simulink model "test1"  (R2020a)
settings: Solver=VariableStepAuto  StartTime=0.0  StopTime=inf  FixedStep=Ts  RelTol=1e-3
PostLoadFcn:
  | , if any(exist('dsrtsu_mdlpostloadfcn', 'file') ~= 0), dsrtsu_mdlpostloadfcn('Execute', bdroot); end,
InitFcn:
  | , if any(exist('rtifpga_mdlclblib', 'file') ~= 0), rtifpga_mdlclblib('Init', bdroot); end,
model workspace (MAT data in the model file):
  FPGA_test1_1_Interrupt_1_1_write : Simulink.Signal (value not decoded)
  FPGA_test1_1_Register_1_1_1_write : Simulink.Signal (value not decoded)
  FPGA_test1_1_Register_2_1_1_write : Simulink.Signal (value not decoded)
  FPGA_test1_1_Register_3_1_1_write : Simulink.Signal (value not decoded)
  FPGA_test1_1_Register_4_1_1_write : Simulink.Signal (value not decoded)
values from neighbouring files (symbols this model uses):
  clamp_threshold = 200    [param.m]
  io_fixed_gain = 10*1000/(3*100)    (= 33.3333333333)    [param.m]
  io_sonda_gain = 10/0.010    (= 1000)    [param.m]
  ioa_gain = 1    [param.m]
  ioa_offset = 0.12    [param.m]
  iob_gain = 1    [param.m]
  iob_offset = 0.06    [param.m]
  ioc_gain = 1    [param.m]
  ioc_offset = -0.1    [param.m]
  Ts = 20e-6    (= 2e-05)    [param.m]
  vclamp_gain = 1010    [param.m]
  vclamp_offset = 10.5    [param.m]
  vi_fixed_gain = 10*44    (= 440)    [param.m]
  vi_sonda_gain = 10*200    (= 2000)    [param.m]
  via_gain = 1    [param.m]
  via_offset = 2.2    [param.m]
  vib_gain = 1    [param.m]
  vib_offset = 3    [param.m]
  vic_gain = 1    [param.m]
  vic_offset = 4.2    [param.m]
libraries: xbsIndex_r4 x428, rti1202lib_adc_class1 x9, rtiproclib x6, simulink x2, rtifpgainterfacelib x1
(part 6 of 7)

== system test1/4_step/FPGA_XDATA_READ_BL1 ==
  CEP1 : xbsIndex_r4/Clock Enable Probe  inherit_constraints=off  block_type=ceprobe
      settings: infoedit="Clock enable extractor.  Produces a Boolean output that mirrors the hardware clock enable associated with the input sample rate.<br><br>Hardware notes: in hardware this block costs nothing."
  CEP3 : xbsIndex_r4/Clock Enable Probe  inherit_constraints=off  block_type=ceprobe
      settings: infoedit="Clock enable extractor.  Produces a Boolean output that mirrors the hardware clock enable associated with the input sample rate.<br><br>Hardware notes: in hardware this block costs nothing."
  Constant1 : xbsIndex_r4/Constant  const=1  gui_display_data_type=Fixed-point  arith_type=Boolean  n_bits=16  bin_pt=14  preci_type=Single  exp_width=8  frac_width=24  explicit_period=on  period=1*1e-08  equ=P=C  opselect=C  inp2=PCIN>>17  opr=+  inp1=P  carry=CIN  dbl_ovrd=off  block_type=constant
  Constant3 : xbsIndex_r4/Constant  const=1  gui_display_data_type=Fixed-point  arith_type=Boolean  n_bits=16  bin_pt=14  preci_type=Single  exp_width=8  frac_width=24  explicit_period=on  period=1*1e-08  equ=P=C  opselect=C  inp2=PCIN>>17  opr=+  inp1=P  carry=CIN  dbl_ovrd=off  block_type=constant
  Delay1 : xbsIndex_r4/Delay  rst=off  infoeditControl=Selection of Reset will increase slice count due to use of real FFs and instead of SRLs  en=off  latency=0  reg_retiming=off  dbl_ovrd=off  block_type=delay
  Delay3 : xbsIndex_r4/Delay  rst=off  infoeditControl=Selection of Reset will increase slice count due to use of real FFs and instead of SRLs  en=off  latency=0  reg_retiming=off  dbl_ovrd=off  block_type=delay
  Register1 : xbsIndex_r4/Register  init=0  rst=off  en=on  dbl_ovrd=off  block_type=register
  Register3 : xbsIndex_r4/Register  init=0  rst=off  en=on  dbl_ovrd=off  block_type=register
  phs_read_register : Subsystem
      mask init:
      | [par, fct] = rtifpgafcnlib('GetCurrentParaValue', get_param(get(gcbh, 'parent'), 'handle'), 'all');
      | if isempty(par) || isempty(fct)
      |     return
      | end
      | binaryPoint = str2double(par(1).Value{1});
      | format = par(2).Value{1};
      | if (strcmp(format, 'signed') == 1)
      |     mode = 0;
      | elseif (strcmp(format, 'unsigned') == 1)
      |     mode = 1;
      | else
      |     % floating-point
      |     mode = 2;
      | end
      | 
      | %Determine PROC sample time
      | proc_sample_time_field = par(5).Value{1};
      | num_val = str2num(proc_sample_time_field);
      | if ~isempty(num_val)
      |     proc_sample_time = num_val;
      | else % search for subsystem/workspace value
      |     proc_sample_time = rtifpgafcnlib('SearchVariableValue', gcbh, proc_sample_time_field);
      |     if ~isnumeric(proc_sample_time)
      |         proc_sample_time = str2double(proc_sample_time);
      |     end
      | end
      | 
      | %Determine FPGA sample rate
      | dataGatewayName = fct.FrameworkIn(1).Name{1};
      | fpga_sample_time = rtifpga_xsgcasinglib('xlGetParam', [gcs '/' dataGatewayName] , 'period');
      | fpga_sample_time = str2double(fpga_sample_time);
  xreg_000_dout : xbsIndex_r4/Gateway In  gui_display_data_type=Fixed-point  arith_type=Unsigned  n_bits=32  bin_pt=0  preci_type=Single  exp_width=8  frac_width=24  rows=1  columns=1  quantization="Round  (unbiased: +/- Inf)"  overflow=Saturate  period=1e-08  UseAsADC=off  ADCChannel='1'  interface=None  automatic_assignment=on  address_offset=hex2dec('00')  intf_name=''  intf_description=''  default_value=0  timing_constraint=None  locs_specified=off  LOCs={}  io_standard={}  inherit_from_input=off  hdl_port=on  dbl_ovrd=off  block_type=gatewayin
  xreg_000_dout_wr : xbsIndex_r4/Gateway In  gui_display_data_type=Fixed-point  arith_type=Unsigned  n_bits=1  bin_pt=0  preci_type=Single  exp_width=8  frac_width=24  rows=1  columns=1  quantization="Round  (unbiased: +/- Inf)"  overflow=Saturate  period=1e-08  UseAsADC=off  ADCChannel='1'  interface=None  automatic_assignment=on  address_offset=hex2dec('00')  intf_name=''  intf_description=''  default_value=0  timing_constraint=None  locs_specified=off  LOCs={}  io_standard={}  inherit_from_input=off  hdl_port=on  dbl_ovrd=off  block_type=gatewayin
  Data : Outport
  Data New : Outport  Port=2
  wires:
  [FPGA_test1_1_Register_1_1_1_write] -> phs_read_register/1(data_i)
  Register1/1 -> Delay1/1
  Delay1/1 -> Data/1
  Constant1/1 -> CEP1/1
  CEP1/1 -> Register1/2
  xreg_000_dout/1 -> Register1/1
  Register3/1 -> Delay3/1
  Delay3/1 -> Data New/1
  Constant3/1 -> CEP3/1
  CEP3/1 -> Register3/2
  xreg_000_dout_wr/1 -> Register3/1
  phs_read_register/1(data_o) -> xreg_000_dout/1
  phs_read_register/2(data_new_o) -> xreg_000_dout_wr/1

== system test1/4_step/FPGA_XDATA_READ_BL2 ==
  CEP1 : xbsIndex_r4/Clock Enable Probe  inherit_constraints=off  block_type=ceprobe
      settings: infoedit="Clock enable extractor.  Produces a Boolean output that mirrors the hardware clock enable associated with the input sample rate.<br><br>Hardware notes: in hardware this block costs nothing."
  CEP3 : xbsIndex_r4/Clock Enable Probe  inherit_constraints=off  block_type=ceprobe
      settings: infoedit="Clock enable extractor.  Produces a Boolean output that mirrors the hardware clock enable associated with the input sample rate.<br><br>Hardware notes: in hardware this block costs nothing."
  Constant1 : xbsIndex_r4/Constant  const=1  gui_display_data_type=Fixed-point  arith_type=Boolean  n_bits=16  bin_pt=14  preci_type=Single  exp_width=8  frac_width=24  explicit_period=on  period=1*1e-08  equ=P=C  opselect=C  inp2=PCIN>>17  opr=+  inp1=P  carry=CIN  dbl_ovrd=off  block_type=constant
  Constant3 : xbsIndex_r4/Constant  const=1  gui_display_data_type=Fixed-point  arith_type=Boolean  n_bits=16  bin_pt=14  preci_type=Single  exp_width=8  frac_width=24  explicit_period=on  period=1*1e-08  equ=P=C  opselect=C  inp2=PCIN>>17  opr=+  inp1=P  carry=CIN  dbl_ovrd=off  block_type=constant
  Delay1 : xbsIndex_r4/Delay  rst=off  infoeditControl=Selection of Reset will increase slice count due to use of real FFs and instead of SRLs  en=off  latency=0  reg_retiming=off  dbl_ovrd=off  block_type=delay
  Delay3 : xbsIndex_r4/Delay  rst=off  infoeditControl=Selection of Reset will increase slice count due to use of real FFs and instead of SRLs  en=off  latency=0  reg_retiming=off  dbl_ovrd=off  block_type=delay
  Register1 : xbsIndex_r4/Register  init=0  rst=off  en=on  dbl_ovrd=off  block_type=register
  Register3 : xbsIndex_r4/Register  init=0  rst=off  en=on  dbl_ovrd=off  block_type=register
  phs_read_register : Subsystem
      mask init: same as test1/4_step/FPGA_XDATA_READ_BL1/phs_read_register
  xreg_001_dout : xbsIndex_r4/Gateway In  gui_display_data_type=Fixed-point  arith_type=Unsigned  n_bits=32  bin_pt=0  preci_type=Single  exp_width=8  frac_width=24  rows=1  columns=1  quantization="Round  (unbiased: +/- Inf)"  overflow=Saturate  period=1e-08  UseAsADC=off  ADCChannel='1'  interface=None  automatic_assignment=on  address_offset=hex2dec('00')  intf_name=''  intf_description=''  default_value=0  timing_constraint=None  locs_specified=off  LOCs={}  io_standard={}  inherit_from_input=off  hdl_port=on  dbl_ovrd=off  block_type=gatewayin
  xreg_001_dout_wr : xbsIndex_r4/Gateway In  gui_display_data_type=Fixed-point  arith_type=Unsigned  n_bits=1  bin_pt=0  preci_type=Single  exp_width=8  frac_width=24  rows=1  columns=1  quantization="Round  (unbiased: +/- Inf)"  overflow=Saturate  period=1e-08  UseAsADC=off  ADCChannel='1'  interface=None  automatic_assignment=on  address_offset=hex2dec('00')  intf_name=''  intf_description=''  default_value=0  timing_constraint=None  locs_specified=off  LOCs={}  io_standard={}  inherit_from_input=off  hdl_port=on  dbl_ovrd=off  block_type=gatewayin
  Data : Outport
  Data New : Outport  Port=2
  wires:
  [FPGA_test1_1_Register_2_1_1_write] -> phs_read_register/1(data_i)
  Register1/1 -> Delay1/1
  Delay1/1 -> Data/1
  Constant1/1 -> CEP1/1
  CEP1/1 -> Register1/2
  xreg_001_dout/1 -> Register1/1
  Register3/1 -> Delay3/1
  Delay3/1 -> Data New/1
  Constant3/1 -> CEP3/1
  CEP3/1 -> Register3/2
  xreg_001_dout_wr/1 -> Register3/1
  phs_read_register/1(data_o) -> xreg_001_dout/1
  phs_read_register/2(data_new_o) -> xreg_001_dout_wr/1

== system test1/4_step/FPGA_XDATA_READ_BL3 ==
  CEP1 : xbsIndex_r4/Clock Enable Probe  inherit_constraints=off  block_type=ceprobe
      settings: infoedit="Clock enable extractor.  Produces a Boolean output that mirrors the hardware clock enable associated with the input sample rate.<br><br>Hardware notes: in hardware this block costs nothing."
  CEP3 : xbsIndex_r4/Clock Enable Probe  inherit_constraints=off  block_type=ceprobe
      settings: infoedit="Clock enable extractor.  Produces a Boolean output that mirrors the hardware clock enable associated with the input sample rate.<br><br>Hardware notes: in hardware this block costs nothing."
  Constant1 : xbsIndex_r4/Constant  const=1  gui_display_data_type=Fixed-point  arith_type=Boolean  n_bits=16  bin_pt=14  preci_type=Single  exp_width=8  frac_width=24  explicit_period=on  period=1*1e-08  equ=P=C  opselect=C  inp2=PCIN>>17  opr=+  inp1=P  carry=CIN  dbl_ovrd=off  block_type=constant
  Constant3 : xbsIndex_r4/Constant  const=1  gui_display_data_type=Fixed-point  arith_type=Boolean  n_bits=16  bin_pt=14  preci_type=Single  exp_width=8  frac_width=24  explicit_period=on  period=1*1e-08  equ=P=C  opselect=C  inp2=PCIN>>17  opr=+  inp1=P  carry=CIN  dbl_ovrd=off  block_type=constant
  Delay1 : xbsIndex_r4/Delay  rst=off  infoeditControl=Selection of Reset will increase slice count due to use of real FFs and instead of SRLs  en=off  latency=0  reg_retiming=off  dbl_ovrd=off  block_type=delay
  Delay3 : xbsIndex_r4/Delay  rst=off  infoeditControl=Selection of Reset will increase slice count due to use of real FFs and instead of SRLs  en=off  latency=0  reg_retiming=off  dbl_ovrd=off  block_type=delay
  Register1 : xbsIndex_r4/Register  init=0  rst=off  en=on  dbl_ovrd=off  block_type=register
  Register3 : xbsIndex_r4/Register  init=0  rst=off  en=on  dbl_ovrd=off  block_type=register
  phs_read_register : Subsystem
      mask init: same as test1/4_step/FPGA_XDATA_READ_BL1/phs_read_register
  xreg_002_dout : xbsIndex_r4/Gateway In  gui_display_data_type=Fixed-point  arith_type=Unsigned  n_bits=32  bin_pt=0  preci_type=Single  exp_width=8  frac_width=24  rows=1  columns=1  quantization="Round  (unbiased: +/- Inf)"  overflow=Saturate  period=1e-08  UseAsADC=off  ADCChannel='1'  interface=None  automatic_assignment=on  address_offset=hex2dec('00')  intf_name=''  intf_description=''  default_value=0  timing_constraint=None  locs_specified=off  LOCs={}  io_standard={}  inherit_from_input=off  hdl_port=on  dbl_ovrd=off  block_type=gatewayin
  xreg_002_dout_wr : xbsIndex_r4/Gateway In  gui_display_data_type=Fixed-point  arith_type=Unsigned  n_bits=1  bin_pt=0  preci_type=Single  exp_width=8  frac_width=24  rows=1  columns=1  quantization="Round  (unbiased: +/- Inf)"  overflow=Saturate  period=1e-08  UseAsADC=off  ADCChannel='1'  interface=None  automatic_assignment=on  address_offset=hex2dec('00')  intf_name=''  intf_description=''  default_value=0  timing_constraint=None  locs_specified=off  LOCs={}  io_standard={}  inherit_from_input=off  hdl_port=on  dbl_ovrd=off  block_type=gatewayin
  Data : Outport
  Data New : Outport  Port=2
  wires:
  [FPGA_test1_1_Register_3_1_1_write] -> phs_read_register/1(data_i)
  Register1/1 -> Delay1/1
  Delay1/1 -> Data/1
  Constant1/1 -> CEP1/1
  CEP1/1 -> Register1/2
  xreg_002_dout/1 -> Register1/1
  Register3/1 -> Delay3/1
  Delay3/1 -> Data New/1
  Constant3/1 -> CEP3/1
  CEP3/1 -> Register3/2
  xreg_002_dout_wr/1 -> Register3/1
  phs_read_register/1(data_o) -> xreg_002_dout/1
  phs_read_register/2(data_new_o) -> xreg_002_dout_wr/1

== system test1/4_step/FPGA_XDATA_READ_BL4 ==
  CEP1 : xbsIndex_r4/Clock Enable Probe  inherit_constraints=off  block_type=ceprobe
      settings: infoedit="Clock enable extractor.  Produces a Boolean output that mirrors the hardware clock enable associated with the input sample rate.<br><br>Hardware notes: in hardware this block costs nothing."
  CEP3 : xbsIndex_r4/Clock Enable Probe  inherit_constraints=off  block_type=ceprobe
      settings: infoedit="Clock enable extractor.  Produces a Boolean output that mirrors the hardware clock enable associated with the input sample rate.<br><br>Hardware notes: in hardware this block costs nothing."
  Constant1 : xbsIndex_r4/Constant  const=1  gui_display_data_type=Fixed-point  arith_type=Boolean  n_bits=16  bin_pt=14  preci_type=Single  exp_width=8  frac_width=24  explicit_period=on  period=1*1e-08  equ=P=C  opselect=C  inp2=PCIN>>17  opr=+  inp1=P  carry=CIN  dbl_ovrd=off  block_type=constant
  Constant3 : xbsIndex_r4/Constant  const=1  gui_display_data_type=Fixed-point  arith_type=Boolean  n_bits=16  bin_pt=14  preci_type=Single  exp_width=8  frac_width=24  explicit_period=on  period=1*1e-08  equ=P=C  opselect=C  inp2=PCIN>>17  opr=+  inp1=P  carry=CIN  dbl_ovrd=off  block_type=constant
  Delay1 : xbsIndex_r4/Delay  rst=off  infoeditControl=Selection of Reset will increase slice count due to use of real FFs and instead of SRLs  en=off  latency=0  reg_retiming=off  dbl_ovrd=off  block_type=delay
  Delay3 : xbsIndex_r4/Delay  rst=off  infoeditControl=Selection of Reset will increase slice count due to use of real FFs and instead of SRLs  en=off  latency=0  reg_retiming=off  dbl_ovrd=off  block_type=delay
  Register1 : xbsIndex_r4/Register  init=0  rst=off  en=on  dbl_ovrd=off  block_type=register
  Register3 : xbsIndex_r4/Register  init=0  rst=off  en=on  dbl_ovrd=off  block_type=register
  phs_read_register : Subsystem
      mask init: same as test1/4_step/FPGA_XDATA_READ_BL1/phs_read_register
  xreg_003_dout : xbsIndex_r4/Gateway In  gui_display_data_type=Fixed-point  arith_type=Unsigned  n_bits=32  bin_pt=0  preci_type=Single  exp_width=8  frac_width=24  rows=1  columns=1  quantization="Round  (unbiased: +/- Inf)"  overflow=Saturate  period=1e-08  UseAsADC=off  ADCChannel='1'  interface=None  automatic_assignment=on  address_offset=hex2dec('00')  intf_name=''  intf_description=''  default_value=0  timing_constraint=None  locs_specified=off  LOCs={}  io_standard={}  inherit_from_input=off  hdl_port=on  dbl_ovrd=off  block_type=gatewayin
  xreg_003_dout_wr : xbsIndex_r4/Gateway In  gui_display_data_type=Fixed-point  arith_type=Unsigned  n_bits=1  bin_pt=0  preci_type=Single  exp_width=8  frac_width=24  rows=1  columns=1  quantization="Round  (unbiased: +/- Inf)"  overflow=Saturate  period=1e-08  UseAsADC=off  ADCChannel='1'  interface=None  automatic_assignment=on  address_offset=hex2dec('00')  intf_name=''  intf_description=''  default_value=0  timing_constraint=None  locs_specified=off  LOCs={}  io_standard={}  inherit_from_input=off  hdl_port=on  dbl_ovrd=off  block_type=gatewayin
  Data : Outport
  Data New : Outport  Port=2
  wires:
  [FPGA_test1_1_Register_4_1_1_write] -> phs_read_register/1(data_i)
  Register1/1 -> Delay1/1
  Delay1/1 -> Data/1
  Constant1/1 -> CEP1/1
  CEP1/1 -> Register1/2
  xreg_003_dout/1 -> Register1/1
  Register3/1 -> Delay3/1
  Delay3/1 -> Data New/1
  Constant3/1 -> CEP3/1
  CEP3/1 -> Register3/2
  xreg_003_dout_wr/1 -> Register3/1
  phs_read_register/1(data_o) -> xreg_003_dout/1
  phs_read_register/2(data_new_o) -> xreg_003_dout_wr/1

== system test1/RTI Data/RTI Data Store ==
  RTI Data Store : Subsystem  mask(RTI_DATA_STORE){}
      mask help:
      | RTI Data Store Block. This block is used by RTI to store internal model dependent data. Deleting this block will result in data loss.
      |
      | NEVER DELETE, COPY, OR MODIFY THIS BLOCK!
      mask Help:
      | RTI Data Store Block. This block is used by RTI to store internal model dependent data. Deleting this block will result in data loss.
      | 
      | NEVER DELETE, COPY, OR MODIFY THIS BLOCK!
      mask Display: text(0.5, 0.5, ' ', 'HorizontalAlignment', 'center');

== system test1/Subsystem/Function-Call Subsystem ==
  iref : Inport
  io : Inport  Port=2
  vi : Inport  Port=3
  T : Inport  Port=4
  function : TriggerPort  TriggerType=function-call  VariantControl=Variant
  MATLAB Function : MATLAB Function  TreatAsAtomicUnit=on
  s : Outport
  wires:
  MATLAB Function/1(y) -> s/1  "s"
  iref/1 -> MATLAB Function/1(iref)
  io/1 -> MATLAB Function/2(io)
  vi/1 -> MATLAB Function/3(vin)
  T/1 -> MATLAB Function/4(T)

== system test1/4_step/FPGA_INT_BL1/phs_interrupt ==
  note: Subsystem simulating the phs bus
      | access via RTLib functions.
  note: Subsystem simulating the communication
      | function specific behaviour. This is how the
      | FPGA framework driver takes effect on the data.
  data_i : Inport
  com_fct_model : Subsystem
  phs/rtlib_sim_model : Subsystem
  data_o : Outport  VectorParamsAs1DForOutWhenUnconnected=off
  wires:
  phs/rtlib_sim_model/1(data_o1) -> data_o/1
  com_fct_model/1(data_o1) -> phs/rtlib_sim_model/1(data_i1)
  data_i/1 -> com_fct_model/1(data_i1)

== system test1/4_step/FPGA_IO_WRITE_BL1/dig_inout_tp1 ==
  note: The nominal input range is NOT simulated because
      | the HW does not saturate according to the input range.
  note: The Digital In value is simulated by Threshold voltage detection.
  data_in_i : Inport
  enable_i : Inport  Port=2
  data_out_i : Inport  Port=3
  direction_i : Inport  Port=4
  Data Type Conversion : DataTypeConversion
  Data Type Conversion1 : DataTypeConversion
  Disabled Input Value : Constant  Value=0
  Disabled Output Value : Constant  Value=0
  Invert : Constant  Value=inverted_dio
  Invert1 : Constant  Value=inverted_dio
  Inverter : Logic  Operator=NOT  AllPortsSameDT=off  OutDataTypeStr=boolean
  Inverter1 : Logic  AllPortsSameDT=off  OutDataTypeStr=boolean
  Inverter2 : Logic  Operator=NOT  AllPortsSameDT=off  OutDataTypeStr=boolean
  Inverter3 : Logic  AllPortsSameDT=off  OutDataTypeStr=boolean
  Inverter4 : Logic  Operator=NOT  AllPortsSameDT=off  OutDataTypeStr=boolean
  Relational Operator : RelationalOperator  OutDataTypeStr=boolean  RndMeth=Nearest
  Switch{,1..3} (4 alike) : Switch  Threshold=1
  Threshold Voltage : Constant  Value=2
  Voltage : Gain  Gain=voltage  ParamDataTypeStr=float('double')
  data_in_o : Outport  VectorParamsAs1DForOutWhenUnconnected=off
  data_out_o : Outport  Port=2  VectorParamsAs1DForOutWhenUnconnected=off
  wires:
  Voltage/1 -> data_out_o/1
  Data Type Conversion1/1 -> Inverter3/2, Inverter2/1
  Data Type Conversion/1 -> Inverter3/1, Inverter1/1
  Switch3/1 -> Voltage/1
  Switch2/1 -> Switch3/3, Inverter4/1
  Inverter4/1 -> Switch3/1
  Invert1/1 -> Switch3/2
  data_out_i/1 -> Switch2/1
  Inverter3/1 -> Switch2/2
  Disabled Output Value/1 -> Switch2/3
  Inverter2/1 -> Inverter1/2
  direction_i/1 -> Data Type Conversion1/1
  Inverter1/1 -> Switch/2
  enable_i/1 -> Data Type Conversion/1
  Switch/1 -> Switch1/3, Inverter/1
  Relational Operator/1 -> Switch/1
  Inverter/1 -> Switch1/1
  Invert/1 -> Switch1/2
  Switch1/1 -> data_in_o/1
  Disabled Input Value/1 -> Switch/3
  Threshold Voltage/1 -> Relational Operator/2
  data_in_i/1 -> Relational Operator/1

== system test1/4_step/FPGA_IO_WRITE_BL10/dig_inout_tp1 ==
  note: The nominal input range is NOT simulated because
      | the HW does not saturate according to the input range.
  note: The Digital In value is simulated by Threshold voltage detection.
  data_in_i : Inport
  enable_i : Inport  Port=2
  data_out_i : Inport  Port=3
  direction_i : Inport  Port=4
  Data Type Conversion : DataTypeConversion
  Data Type Conversion1 : DataTypeConversion
  Disabled Input Value : Constant  Value=0
  Disabled Output Value : Constant  Value=0
  Invert : Constant  Value=inverted_dio
  Invert1 : Constant  Value=inverted_dio
  Inverter : Logic  Operator=NOT  AllPortsSameDT=off  OutDataTypeStr=boolean
  Inverter1 : Logic  AllPortsSameDT=off  OutDataTypeStr=boolean
  Inverter2 : Logic  Operator=NOT  AllPortsSameDT=off  OutDataTypeStr=boolean
  Inverter3 : Logic  AllPortsSameDT=off  OutDataTypeStr=boolean
  Inverter4 : Logic  Operator=NOT  AllPortsSameDT=off  OutDataTypeStr=boolean
  Relational Operator : RelationalOperator  OutDataTypeStr=boolean  RndMeth=Nearest
  Switch{,1..3} (4 alike) : Switch  Threshold=1
  Threshold Voltage : Constant  Value=2
  Voltage : Gain  Gain=voltage  ParamDataTypeStr=float('double')
  data_in_o : Outport  VectorParamsAs1DForOutWhenUnconnected=off
  data_out_o : Outport  Port=2  VectorParamsAs1DForOutWhenUnconnected=off
  wires:
  Voltage/1 -> data_out_o/1
  Data Type Conversion1/1 -> Inverter3/2, Inverter2/1
  Data Type Conversion/1 -> Inverter3/1, Inverter1/1
  Switch3/1 -> Voltage/1
  Switch2/1 -> Switch3/3, Inverter4/1
  Inverter4/1 -> Switch3/1
  Invert1/1 -> Switch3/2
  data_out_i/1 -> Switch2/1
  Inverter3/1 -> Switch2/2
  Disabled Output Value/1 -> Switch2/3
  Inverter2/1 -> Inverter1/2
  direction_i/1 -> Data Type Conversion1/1
  Inverter1/1 -> Switch/2
  enable_i/1 -> Data Type Conversion/1
  Switch/1 -> Switch1/3, Inverter/1
  Relational Operator/1 -> Switch/1
  Inverter/1 -> Switch1/1
  Invert/1 -> Switch1/2
  Switch1/1 -> data_in_o/1
  Disabled Input Value/1 -> Switch/3
  Threshold Voltage/1 -> Relational Operator/2
  data_in_i/1 -> Relational Operator/1

== system test1/4_step/FPGA_IO_WRITE_BL11/dig_inout_tp1 ==
  note: The nominal input range is NOT simulated because
      | the HW does not saturate according to the input range.
  note: The Digital In value is simulated by Threshold voltage detection.
  data_in_i : Inport
  enable_i : Inport  Port=2
  data_out_i : Inport  Port=3
  direction_i : Inport  Port=4
  Data Type Conversion : DataTypeConversion
  Data Type Conversion1 : DataTypeConversion
  Disabled Input Value : Constant  Value=0
  Disabled Output Value : Constant  Value=0
  Invert : Constant  Value=inverted_dio
  Invert1 : Constant  Value=inverted_dio
  Inverter : Logic  Operator=NOT  AllPortsSameDT=off  OutDataTypeStr=boolean
  Inverter1 : Logic  AllPortsSameDT=off  OutDataTypeStr=boolean
  Inverter2 : Logic  Operator=NOT  AllPortsSameDT=off  OutDataTypeStr=boolean
  Inverter3 : Logic  AllPortsSameDT=off  OutDataTypeStr=boolean
  Inverter4 : Logic  Operator=NOT  AllPortsSameDT=off  OutDataTypeStr=boolean
  Relational Operator : RelationalOperator  OutDataTypeStr=boolean  RndMeth=Nearest
  Switch{,1..3} (4 alike) : Switch  Threshold=1
  Threshold Voltage : Constant  Value=2
  Voltage : Gain  Gain=voltage  ParamDataTypeStr=float('double')
  data_in_o : Outport  VectorParamsAs1DForOutWhenUnconnected=off
  data_out_o : Outport  Port=2  VectorParamsAs1DForOutWhenUnconnected=off
  wires:
  Voltage/1 -> data_out_o/1
  Data Type Conversion1/1 -> Inverter3/2, Inverter2/1
  Data Type Conversion/1 -> Inverter3/1, Inverter1/1
  Switch3/1 -> Voltage/1
  Switch2/1 -> Switch3/3, Inverter4/1
  Inverter4/1 -> Switch3/1
  Invert1/1 -> Switch3/2
  data_out_i/1 -> Switch2/1
  Inverter3/1 -> Switch2/2
  Disabled Output Value/1 -> Switch2/3
  Inverter2/1 -> Inverter1/2
  direction_i/1 -> Data Type Conversion1/1
  Inverter1/1 -> Switch/2
  enable_i/1 -> Data Type Conversion/1
  Switch/1 -> Switch1/3, Inverter/1
  Relational Operator/1 -> Switch/1
  Inverter/1 -> Switch1/1
  Invert/1 -> Switch1/2
  Switch1/1 -> data_in_o/1
  Disabled Input Value/1 -> Switch/3
  Threshold Voltage/1 -> Relational Operator/2
  data_in_i/1 -> Relational Operator/1

== system test1/4_step/FPGA_IO_WRITE_BL12/dig_inout_tp1 ==
  note: The nominal input range is NOT simulated because
      | the HW does not saturate according to the input range.
  note: The Digital In value is simulated by Threshold voltage detection.
  data_in_i : Inport
  enable_i : Inport  Port=2
  data_out_i : Inport  Port=3
  direction_i : Inport  Port=4
  Data Type Conversion : DataTypeConversion
  Data Type Conversion1 : DataTypeConversion
  Disabled Input Value : Constant  Value=0
  Disabled Output Value : Constant  Value=0
  Invert : Constant  Value=inverted_dio
  Invert1 : Constant  Value=inverted_dio
  Inverter : Logic  Operator=NOT  AllPortsSameDT=off  OutDataTypeStr=boolean
  Inverter1 : Logic  AllPortsSameDT=off  OutDataTypeStr=boolean
  Inverter2 : Logic  Operator=NOT  AllPortsSameDT=off  OutDataTypeStr=boolean
  Inverter3 : Logic  AllPortsSameDT=off  OutDataTypeStr=boolean
  Inverter4 : Logic  Operator=NOT  AllPortsSameDT=off  OutDataTypeStr=boolean
  Relational Operator : RelationalOperator  OutDataTypeStr=boolean  RndMeth=Nearest
  Switch{,1..3} (4 alike) : Switch  Threshold=1
  Threshold Voltage : Constant  Value=2
  Voltage : Gain  Gain=voltage  ParamDataTypeStr=float('double')
  data_in_o : Outport  VectorParamsAs1DForOutWhenUnconnected=off
  data_out_o : Outport  Port=2  VectorParamsAs1DForOutWhenUnconnected=off
  wires:
  Voltage/1 -> data_out_o/1
  Data Type Conversion1/1 -> Inverter3/2, Inverter2/1
  Data Type Conversion/1 -> Inverter3/1, Inverter1/1
  Switch3/1 -> Voltage/1
  Switch2/1 -> Switch3/3, Inverter4/1
  Inverter4/1 -> Switch3/1
  Invert1/1 -> Switch3/2
  data_out_i/1 -> Switch2/1
  Inverter3/1 -> Switch2/2
  Disabled Output Value/1 -> Switch2/3
  Inverter2/1 -> Inverter1/2
  direction_i/1 -> Data Type Conversion1/1
  Inverter1/1 -> Switch/2
  enable_i/1 -> Data Type Conversion/1
  Switch/1 -> Switch1/3, Inverter/1
  Relational Operator/1 -> Switch/1
  Inverter/1 -> Switch1/1
  Invert/1 -> Switch1/2
  Switch1/1 -> data_in_o/1
  Disabled Input Value/1 -> Switch/3
  Threshold Voltage/1 -> Relational Operator/2
  data_in_i/1 -> Relational Operator/1

== system test1/4_step/FPGA_IO_WRITE_BL13/dig_inout_tp1 ==
  note: The nominal input range is NOT simulated because
      | the HW does not saturate according to the input range.
  note: The Digital In value is simulated by Threshold voltage detection.
  data_in_i : Inport
  enable_i : Inport  Port=2
  data_out_i : Inport  Port=3
  direction_i : Inport  Port=4
  Data Type Conversion : DataTypeConversion
  Data Type Conversion1 : DataTypeConversion
  Disabled Input Value : Constant  Value=0
  Disabled Output Value : Constant  Value=0
  Invert : Constant  Value=inverted_dio
  Invert1 : Constant  Value=inverted_dio
  Inverter : Logic  Operator=NOT  AllPortsSameDT=off  OutDataTypeStr=boolean
  Inverter1 : Logic  AllPortsSameDT=off  OutDataTypeStr=boolean
  Inverter2 : Logic  Operator=NOT  AllPortsSameDT=off  OutDataTypeStr=boolean
  Inverter3 : Logic  AllPortsSameDT=off  OutDataTypeStr=boolean
  Inverter4 : Logic  Operator=NOT  AllPortsSameDT=off  OutDataTypeStr=boolean
  Relational Operator : RelationalOperator  OutDataTypeStr=boolean  RndMeth=Nearest
  Switch{,1..3} (4 alike) : Switch  Threshold=1
  Threshold Voltage : Constant  Value=2
  Voltage : Gain  Gain=voltage  ParamDataTypeStr=float('double')
  data_in_o : Outport  VectorParamsAs1DForOutWhenUnconnected=off
  data_out_o : Outport  Port=2  VectorParamsAs1DForOutWhenUnconnected=off
  wires:
  Voltage/1 -> data_out_o/1
  Data Type Conversion1/1 -> Inverter3/2, Inverter2/1
  Data Type Conversion/1 -> Inverter3/1, Inverter1/1
  Switch3/1 -> Voltage/1
  Switch2/1 -> Switch3/3, Inverter4/1
  Inverter4/1 -> Switch3/1
  Invert1/1 -> Switch3/2
  data_out_i/1 -> Switch2/1
  Inverter3/1 -> Switch2/2
  Disabled Output Value/1 -> Switch2/3
  Inverter2/1 -> Inverter1/2
  direction_i/1 -> Data Type Conversion1/1
  Inverter1/1 -> Switch/2
  enable_i/1 -> Data Type Conversion/1
  Switch/1 -> Switch1/3, Inverter/1
  Relational Operator/1 -> Switch/1
  Inverter/1 -> Switch1/1
  Invert/1 -> Switch1/2
  Switch1/1 -> data_in_o/1
  Disabled Input Value/1 -> Switch/3
  Threshold Voltage/1 -> Relational Operator/2
  data_in_i/1 -> Relational Operator/1

== system test1/4_step/FPGA_IO_WRITE_BL14/dig_inout_tp1 ==
  note: The nominal input range is NOT simulated because
      | the HW does not saturate according to the input range.
  note: The Digital In value is simulated by Threshold voltage detection.
  data_in_i : Inport
  enable_i : Inport  Port=2
  data_out_i : Inport  Port=3
  direction_i : Inport  Port=4
  Data Type Conversion : DataTypeConversion
  Data Type Conversion1 : DataTypeConversion
  Disabled Input Value : Constant  Value=0
  Disabled Output Value : Constant  Value=0
  Invert : Constant  Value=inverted_dio
  Invert1 : Constant  Value=inverted_dio
  Inverter : Logic  Operator=NOT  AllPortsSameDT=off  OutDataTypeStr=boolean
  Inverter1 : Logic  AllPortsSameDT=off  OutDataTypeStr=boolean
  Inverter2 : Logic  Operator=NOT  AllPortsSameDT=off  OutDataTypeStr=boolean
  Inverter3 : Logic  AllPortsSameDT=off  OutDataTypeStr=boolean
  Inverter4 : Logic  Operator=NOT  AllPortsSameDT=off  OutDataTypeStr=boolean
  Relational Operator : RelationalOperator  OutDataTypeStr=boolean  RndMeth=Nearest
  Switch{,1..3} (4 alike) : Switch  Threshold=1
  Threshold Voltage : Constant  Value=2
  Voltage : Gain  Gain=voltage  ParamDataTypeStr=float('double')
  data_in_o : Outport  VectorParamsAs1DForOutWhenUnconnected=off
  data_out_o : Outport  Port=2  VectorParamsAs1DForOutWhenUnconnected=off
  wires:
  Voltage/1 -> data_out_o/1
  Data Type Conversion1/1 -> Inverter3/2, Inverter2/1
  Data Type Conversion/1 -> Inverter3/1, Inverter1/1
  Switch3/1 -> Voltage/1
  Switch2/1 -> Switch3/3, Inverter4/1
  Inverter4/1 -> Switch3/1
  Invert1/1 -> Switch3/2
  data_out_i/1 -> Switch2/1
  Inverter3/1 -> Switch2/2
  Disabled Output Value/1 -> Switch2/3
  Inverter2/1 -> Inverter1/2
  direction_i/1 -> Data Type Conversion1/1
  Inverter1/1 -> Switch/2
  enable_i/1 -> Data Type Conversion/1
  Switch/1 -> Switch1/3, Inverter/1
  Relational Operator/1 -> Switch/1
  Inverter/1 -> Switch1/1
  Invert/1 -> Switch1/2
  Switch1/1 -> data_in_o/1
  Disabled Input Value/1 -> Switch/3
  Threshold Voltage/1 -> Relational Operator/2
  data_in_i/1 -> Relational Operator/1

== system test1/4_step/FPGA_IO_WRITE_BL15/dig_inout_tp1 ==
  note: The nominal input range is NOT simulated because
      | the HW does not saturate according to the input range.
  note: The Digital In value is simulated by Threshold voltage detection.
  data_in_i : Inport
  enable_i : Inport  Port=2
  data_out_i : Inport  Port=3
  direction_i : Inport  Port=4
  Data Type Conversion : DataTypeConversion
  Data Type Conversion1 : DataTypeConversion
  Disabled Input Value : Constant  Value=0
  Disabled Output Value : Constant  Value=0
  Invert : Constant  Value=inverted_dio
  Invert1 : Constant  Value=inverted_dio
  Inverter : Logic  Operator=NOT  AllPortsSameDT=off  OutDataTypeStr=boolean
  Inverter1 : Logic  AllPortsSameDT=off  OutDataTypeStr=boolean
  Inverter2 : Logic  Operator=NOT  AllPortsSameDT=off  OutDataTypeStr=boolean
  Inverter3 : Logic  AllPortsSameDT=off  OutDataTypeStr=boolean
  Inverter4 : Logic  Operator=NOT  AllPortsSameDT=off  OutDataTypeStr=boolean
  Relational Operator : RelationalOperator  OutDataTypeStr=boolean  RndMeth=Nearest
  Switch{,1..3} (4 alike) : Switch  Threshold=1
  Threshold Voltage : Constant  Value=2
  Voltage : Gain  Gain=voltage  ParamDataTypeStr=float('double')
  data_in_o : Outport  VectorParamsAs1DForOutWhenUnconnected=off
  data_out_o : Outport  Port=2  VectorParamsAs1DForOutWhenUnconnected=off
  wires:
  Voltage/1 -> data_out_o/1
  Data Type Conversion1/1 -> Inverter3/2, Inverter2/1
  Data Type Conversion/1 -> Inverter3/1, Inverter1/1
  Switch3/1 -> Voltage/1
  Switch2/1 -> Switch3/3, Inverter4/1
  Inverter4/1 -> Switch3/1
  Invert1/1 -> Switch3/2
  data_out_i/1 -> Switch2/1
  Inverter3/1 -> Switch2/2
  Disabled Output Value/1 -> Switch2/3
  Inverter2/1 -> Inverter1/2
  direction_i/1 -> Data Type Conversion1/1
  Inverter1/1 -> Switch/2
  enable_i/1 -> Data Type Conversion/1
  Switch/1 -> Switch1/3, Inverter/1
  Relational Operator/1 -> Switch/1
  Inverter/1 -> Switch1/1
  Invert/1 -> Switch1/2
  Switch1/1 -> data_in_o/1
  Disabled Input Value/1 -> Switch/3
  Threshold Voltage/1 -> Relational Operator/2
  data_in_i/1 -> Relational Operator/1

== system test1/4_step/FPGA_IO_WRITE_BL16/dig_inout_tp1 ==
  note: The nominal input range is NOT simulated because
      | the HW does not saturate according to the input range.
  note: The Digital In value is simulated by Threshold voltage detection.
  data_in_i : Inport
  enable_i : Inport  Port=2
  data_out_i : Inport  Port=3
  direction_i : Inport  Port=4
  Data Type Conversion : DataTypeConversion
  Data Type Conversion1 : DataTypeConversion
  Disabled Input Value : Constant  Value=0
  Disabled Output Value : Constant  Value=0
  Invert : Constant  Value=inverted_dio
  Invert1 : Constant  Value=inverted_dio
  Inverter : Logic  Operator=NOT  AllPortsSameDT=off  OutDataTypeStr=boolean
  Inverter1 : Logic  AllPortsSameDT=off  OutDataTypeStr=boolean
  Inverter2 : Logic  Operator=NOT  AllPortsSameDT=off  OutDataTypeStr=boolean
  Inverter3 : Logic  AllPortsSameDT=off  OutDataTypeStr=boolean
  Inverter4 : Logic  Operator=NOT  AllPortsSameDT=off  OutDataTypeStr=boolean
  Relational Operator : RelationalOperator  OutDataTypeStr=boolean  RndMeth=Nearest
  Switch{,1..3} (4 alike) : Switch  Threshold=1
  Threshold Voltage : Constant  Value=2
  Voltage : Gain  Gain=voltage  ParamDataTypeStr=float('double')
  data_in_o : Outport  VectorParamsAs1DForOutWhenUnconnected=off
  data_out_o : Outport  Port=2  VectorParamsAs1DForOutWhenUnconnected=off
  wires:
  Voltage/1 -> data_out_o/1
  Data Type Conversion1/1 -> Inverter3/2, Inverter2/1
  Data Type Conversion/1 -> Inverter3/1, Inverter1/1
  Switch3/1 -> Voltage/1
  Switch2/1 -> Switch3/3, Inverter4/1
  Inverter4/1 -> Switch3/1
  Invert1/1 -> Switch3/2
  data_out_i/1 -> Switch2/1
  Inverter3/1 -> Switch2/2
  Disabled Output Value/1 -> Switch2/3
  Inverter2/1 -> Inverter1/2
  direction_i/1 -> Data Type Conversion1/1
  Inverter1/1 -> Switch/2
  enable_i/1 -> Data Type Conversion/1
  Switch/1 -> Switch1/3, Inverter/1
  Relational Operator/1 -> Switch/1
  Inverter/1 -> Switch1/1
  Invert/1 -> Switch1/2
  Switch1/1 -> data_in_o/1
  Disabled Input Value/1 -> Switch/3
  Threshold Voltage/1 -> Relational Operator/2
  data_in_i/1 -> Relational Operator/1

== system test1/4_step/FPGA_IO_WRITE_BL17/dig_inout_tp1 ==
  note: The nominal input range is NOT simulated because
      | the HW does not saturate according to the input range.
  note: The Digital In value is simulated by Threshold voltage detection.
  data_in_i : Inport
  enable_i : Inport  Port=2
  data_out_i : Inport  Port=3
  direction_i : Inport  Port=4
  Data Type Conversion : DataTypeConversion
  Data Type Conversion1 : DataTypeConversion
  Disabled Input Value : Constant  Value=0
  Disabled Output Value : Constant  Value=0
  Invert : Constant  Value=inverted_dio
  Invert1 : Constant  Value=inverted_dio
  Inverter : Logic  Operator=NOT  AllPortsSameDT=off  OutDataTypeStr=boolean
  Inverter1 : Logic  AllPortsSameDT=off  OutDataTypeStr=boolean
  Inverter2 : Logic  Operator=NOT  AllPortsSameDT=off  OutDataTypeStr=boolean
  Inverter3 : Logic  AllPortsSameDT=off  OutDataTypeStr=boolean
  Inverter4 : Logic  Operator=NOT  AllPortsSameDT=off  OutDataTypeStr=boolean
  Relational Operator : RelationalOperator  OutDataTypeStr=boolean  RndMeth=Nearest
  Switch{,1..3} (4 alike) : Switch  Threshold=1
  Threshold Voltage : Constant  Value=2
  Voltage : Gain  Gain=voltage  ParamDataTypeStr=float('double')
  data_in_o : Outport  VectorParamsAs1DForOutWhenUnconnected=off
  data_out_o : Outport  Port=2  VectorParamsAs1DForOutWhenUnconnected=off
  wires:
  Voltage/1 -> data_out_o/1
  Data Type Conversion1/1 -> Inverter3/2, Inverter2/1
  Data Type Conversion/1 -> Inverter3/1, Inverter1/1
  Switch3/1 -> Voltage/1
  Switch2/1 -> Switch3/3, Inverter4/1
  Inverter4/1 -> Switch3/1
  Invert1/1 -> Switch3/2
  data_out_i/1 -> Switch2/1
  Inverter3/1 -> Switch2/2
  Disabled Output Value/1 -> Switch2/3
  Inverter2/1 -> Inverter1/2
  direction_i/1 -> Data Type Conversion1/1
  Inverter1/1 -> Switch/2
  enable_i/1 -> Data Type Conversion/1
  Switch/1 -> Switch1/3, Inverter/1
  Relational Operator/1 -> Switch/1
  Inverter/1 -> Switch1/1
  Invert/1 -> Switch1/2
  Switch1/1 -> data_in_o/1
  Disabled Input Value/1 -> Switch/3
  Threshold Voltage/1 -> Relational Operator/2
  data_in_i/1 -> Relational Operator/1

== system test1/4_step/FPGA_IO_WRITE_BL18/dig_inout_tp1 ==
  note: The nominal input range is NOT simulated because
      | the HW does not saturate according to the input range.
  note: The Digital In value is simulated by Threshold voltage detection.
  data_in_i : Inport
  enable_i : Inport  Port=2
  data_out_i : Inport  Port=3
  direction_i : Inport  Port=4
  Data Type Conversion : DataTypeConversion
  Data Type Conversion1 : DataTypeConversion
  Disabled Input Value : Constant  Value=0
  Disabled Output Value : Constant  Value=0
  Invert : Constant  Value=inverted_dio
  Invert1 : Constant  Value=inverted_dio
  Inverter : Logic  Operator=NOT  AllPortsSameDT=off  OutDataTypeStr=boolean
  Inverter1 : Logic  AllPortsSameDT=off  OutDataTypeStr=boolean
  Inverter2 : Logic  Operator=NOT  AllPortsSameDT=off  OutDataTypeStr=boolean
  Inverter3 : Logic  AllPortsSameDT=off  OutDataTypeStr=boolean
  Inverter4 : Logic  Operator=NOT  AllPortsSameDT=off  OutDataTypeStr=boolean
  Relational Operator : RelationalOperator  OutDataTypeStr=boolean  RndMeth=Nearest
  Switch{,1..3} (4 alike) : Switch  Threshold=1
  Threshold Voltage : Constant  Value=2
  Voltage : Gain  Gain=voltage  ParamDataTypeStr=float('double')
  data_in_o : Outport  VectorParamsAs1DForOutWhenUnconnected=off
  data_out_o : Outport  Port=2  VectorParamsAs1DForOutWhenUnconnected=off
  wires:
  Voltage/1 -> data_out_o/1
  Data Type Conversion1/1 -> Inverter3/2, Inverter2/1
  Data Type Conversion/1 -> Inverter3/1, Inverter1/1
  Switch3/1 -> Voltage/1
  Switch2/1 -> Switch3/3, Inverter4/1
  Inverter4/1 -> Switch3/1
  Invert1/1 -> Switch3/2
  data_out_i/1 -> Switch2/1
  Inverter3/1 -> Switch2/2
  Disabled Output Value/1 -> Switch2/3
  Inverter2/1 -> Inverter1/2
  direction_i/1 -> Data Type Conversion1/1
  Inverter1/1 -> Switch/2
  enable_i/1 -> Data Type Conversion/1
  Switch/1 -> Switch1/3, Inverter/1
  Relational Operator/1 -> Switch/1
  Inverter/1 -> Switch1/1
  Invert/1 -> Switch1/2
  Switch1/1 -> data_in_o/1
  Disabled Input Value/1 -> Switch/3
  Threshold Voltage/1 -> Relational Operator/2
  data_in_i/1 -> Relational Operator/1

== system test1/4_step/FPGA_IO_WRITE_BL2/dig_inout_tp1 ==
  note: The nominal input range is NOT simulated because
      | the HW does not saturate according to the input range.
  note: The Digital In value is simulated by Threshold voltage detection.
  data_in_i : Inport
  enable_i : Inport  Port=2
  data_out_i : Inport  Port=3
  direction_i : Inport  Port=4
  Data Type Conversion : DataTypeConversion
  Data Type Conversion1 : DataTypeConversion
  Disabled Input Value : Constant  Value=0
  Disabled Output Value : Constant  Value=0
  Invert : Constant  Value=inverted_dio
  Invert1 : Constant  Value=inverted_dio
  Inverter : Logic  Operator=NOT  AllPortsSameDT=off  OutDataTypeStr=boolean
  Inverter1 : Logic  AllPortsSameDT=off  OutDataTypeStr=boolean
  Inverter2 : Logic  Operator=NOT  AllPortsSameDT=off  OutDataTypeStr=boolean
  Inverter3 : Logic  AllPortsSameDT=off  OutDataTypeStr=boolean
  Inverter4 : Logic  Operator=NOT  AllPortsSameDT=off  OutDataTypeStr=boolean
  Relational Operator : RelationalOperator  OutDataTypeStr=boolean  RndMeth=Nearest
  Switch{,1..3} (4 alike) : Switch  Threshold=1
  Threshold Voltage : Constant  Value=2
  Voltage : Gain  Gain=voltage  ParamDataTypeStr=float('double')
  data_in_o : Outport  VectorParamsAs1DForOutWhenUnconnected=off
  data_out_o : Outport  Port=2  VectorParamsAs1DForOutWhenUnconnected=off
  wires:
  Voltage/1 -> data_out_o/1
  Data Type Conversion1/1 -> Inverter3/2, Inverter2/1
  Data Type Conversion/1 -> Inverter3/1, Inverter1/1
  Switch3/1 -> Voltage/1
  Switch2/1 -> Switch3/3, Inverter4/1
  Inverter4/1 -> Switch3/1
  Invert1/1 -> Switch3/2
  data_out_i/1 -> Switch2/1
  Inverter3/1 -> Switch2/2
  Disabled Output Value/1 -> Switch2/3
  Inverter2/1 -> Inverter1/2
  direction_i/1 -> Data Type Conversion1/1
  Inverter1/1 -> Switch/2
  enable_i/1 -> Data Type Conversion/1
  Switch/1 -> Switch1/3, Inverter/1
  Relational Operator/1 -> Switch/1
  Inverter/1 -> Switch1/1
  Invert/1 -> Switch1/2
  Switch1/1 -> data_in_o/1
  Disabled Input Value/1 -> Switch/3
  Threshold Voltage/1 -> Relational Operator/2
  data_in_i/1 -> Relational Operator/1

== system test1/4_step/FPGA_IO_WRITE_BL3/dig_inout_tp1 ==
  note: The nominal input range is NOT simulated because
      | the HW does not saturate according to the input range.
  note: The Digital In value is simulated by Threshold voltage detection.
  data_in_i : Inport
  enable_i : Inport  Port=2
  data_out_i : Inport  Port=3
  direction_i : Inport  Port=4
  Data Type Conversion : DataTypeConversion
  Data Type Conversion1 : DataTypeConversion
  Disabled Input Value : Constant  Value=0
  Disabled Output Value : Constant  Value=0
  Invert : Constant  Value=inverted_dio
  Invert1 : Constant  Value=inverted_dio
  Inverter : Logic  Operator=NOT  AllPortsSameDT=off  OutDataTypeStr=boolean
  Inverter1 : Logic  AllPortsSameDT=off  OutDataTypeStr=boolean
  Inverter2 : Logic  Operator=NOT  AllPortsSameDT=off  OutDataTypeStr=boolean
  Inverter3 : Logic  AllPortsSameDT=off  OutDataTypeStr=boolean
  Inverter4 : Logic  Operator=NOT  AllPortsSameDT=off  OutDataTypeStr=boolean
  Relational Operator : RelationalOperator  OutDataTypeStr=boolean  RndMeth=Nearest
  Switch{,1..3} (4 alike) : Switch  Threshold=1
  Threshold Voltage : Constant  Value=2
  Voltage : Gain  Gain=voltage  ParamDataTypeStr=float('double')
  data_in_o : Outport  VectorParamsAs1DForOutWhenUnconnected=off
  data_out_o : Outport  Port=2  VectorParamsAs1DForOutWhenUnconnected=off
  wires:
  Voltage/1 -> data_out_o/1
  Data Type Conversion1/1 -> Inverter3/2, Inverter2/1
  Data Type Conversion/1 -> Inverter3/1, Inverter1/1
  Switch3/1 -> Voltage/1
  Switch2/1 -> Switch3/3, Inverter4/1
  Inverter4/1 -> Switch3/1
  Invert1/1 -> Switch3/2
  data_out_i/1 -> Switch2/1
  Inverter3/1 -> Switch2/2
  Disabled Output Value/1 -> Switch2/3
  Inverter2/1 -> Inverter1/2
  direction_i/1 -> Data Type Conversion1/1
  Inverter1/1 -> Switch/2
  enable_i/1 -> Data Type Conversion/1
  Switch/1 -> Switch1/3, Inverter/1
  Relational Operator/1 -> Switch/1
  Inverter/1 -> Switch1/1
  Invert/1 -> Switch1/2
  Switch1/1 -> data_in_o/1
  Disabled Input Value/1 -> Switch/3
  Threshold Voltage/1 -> Relational Operator/2
  data_in_i/1 -> Relational Operator/1

== system test1/4_step/FPGA_IO_WRITE_BL4/dig_inout_tp1 ==
  note: The nominal input range is NOT simulated because
      | the HW does not saturate according to the input range.
  note: The Digital In value is simulated by Threshold voltage detection.
  data_in_i : Inport
  enable_i : Inport  Port=2
  data_out_i : Inport  Port=3
  direction_i : Inport  Port=4
  Data Type Conversion : DataTypeConversion
  Data Type Conversion1 : DataTypeConversion
  Disabled Input Value : Constant  Value=0
  Disabled Output Value : Constant  Value=0
  Invert : Constant  Value=inverted_dio
  Invert1 : Constant  Value=inverted_dio
  Inverter : Logic  Operator=NOT  AllPortsSameDT=off  OutDataTypeStr=boolean
  Inverter1 : Logic  AllPortsSameDT=off  OutDataTypeStr=boolean
  Inverter2 : Logic  Operator=NOT  AllPortsSameDT=off  OutDataTypeStr=boolean
  Inverter3 : Logic  AllPortsSameDT=off  OutDataTypeStr=boolean
  Inverter4 : Logic  Operator=NOT  AllPortsSameDT=off  OutDataTypeStr=boolean
  Relational Operator : RelationalOperator  OutDataTypeStr=boolean  RndMeth=Nearest
  Switch{,1..3} (4 alike) : Switch  Threshold=1
  Threshold Voltage : Constant  Value=2
  Voltage : Gain  Gain=voltage  ParamDataTypeStr=float('double')
  data_in_o : Outport  VectorParamsAs1DForOutWhenUnconnected=off
  data_out_o : Outport  Port=2  VectorParamsAs1DForOutWhenUnconnected=off
  wires:
  Voltage/1 -> data_out_o/1
  Data Type Conversion1/1 -> Inverter3/2, Inverter2/1
  Data Type Conversion/1 -> Inverter3/1, Inverter1/1
  Switch3/1 -> Voltage/1
  Switch2/1 -> Switch3/3, Inverter4/1
  Inverter4/1 -> Switch3/1
  Invert1/1 -> Switch3/2
  data_out_i/1 -> Switch2/1
  Inverter3/1 -> Switch2/2
  Disabled Output Value/1 -> Switch2/3
  Inverter2/1 -> Inverter1/2
  direction_i/1 -> Data Type Conversion1/1
  Inverter1/1 -> Switch/2
  enable_i/1 -> Data Type Conversion/1
  Switch/1 -> Switch1/3, Inverter/1
  Relational Operator/1 -> Switch/1
  Inverter/1 -> Switch1/1
  Invert/1 -> Switch1/2
  Switch1/1 -> data_in_o/1
  Disabled Input Value/1 -> Switch/3
  Threshold Voltage/1 -> Relational Operator/2
  data_in_i/1 -> Relational Operator/1

== system test1/4_step/FPGA_IO_WRITE_BL5/dig_inout_tp1 ==
  note: The nominal input range is NOT simulated because
      | the HW does not saturate according to the input range.
  note: The Digital In value is simulated by Threshold voltage detection.
  data_in_i : Inport
  enable_i : Inport  Port=2
  data_out_i : Inport  Port=3
  direction_i : Inport  Port=4
  Data Type Conversion : DataTypeConversion
  Data Type Conversion1 : DataTypeConversion
  Disabled Input Value : Constant  Value=0
  Disabled Output Value : Constant  Value=0
  Invert : Constant  Value=inverted_dio
  Invert1 : Constant  Value=inverted_dio
  Inverter : Logic  Operator=NOT  AllPortsSameDT=off  OutDataTypeStr=boolean
  Inverter1 : Logic  AllPortsSameDT=off  OutDataTypeStr=boolean
  Inverter2 : Logic  Operator=NOT  AllPortsSameDT=off  OutDataTypeStr=boolean
  Inverter3 : Logic  AllPortsSameDT=off  OutDataTypeStr=boolean
  Inverter4 : Logic  Operator=NOT  AllPortsSameDT=off  OutDataTypeStr=boolean
  Relational Operator : RelationalOperator  OutDataTypeStr=boolean  RndMeth=Nearest
  Switch{,1..3} (4 alike) : Switch  Threshold=1
  Threshold Voltage : Constant  Value=2
  Voltage : Gain  Gain=voltage  ParamDataTypeStr=float('double')
  data_in_o : Outport  VectorParamsAs1DForOutWhenUnconnected=off
  data_out_o : Outport  Port=2  VectorParamsAs1DForOutWhenUnconnected=off
  wires:
  Voltage/1 -> data_out_o/1
  Data Type Conversion1/1 -> Inverter3/2, Inverter2/1
  Data Type Conversion/1 -> Inverter3/1, Inverter1/1
  Switch3/1 -> Voltage/1
  Switch2/1 -> Switch3/3, Inverter4/1
  Inverter4/1 -> Switch3/1
  Invert1/1 -> Switch3/2
  data_out_i/1 -> Switch2/1
  Inverter3/1 -> Switch2/2
  Disabled Output Value/1 -> Switch2/3
  Inverter2/1 -> Inverter1/2
  direction_i/1 -> Data Type Conversion1/1
  Inverter1/1 -> Switch/2
  enable_i/1 -> Data Type Conversion/1
  Switch/1 -> Switch1/3, Inverter/1
  Relational Operator/1 -> Switch/1
  Inverter/1 -> Switch1/1
  Invert/1 -> Switch1/2
  Switch1/1 -> data_in_o/1
  Disabled Input Value/1 -> Switch/3
  Threshold Voltage/1 -> Relational Operator/2
  data_in_i/1 -> Relational Operator/1
